simulink model "exercise22_05_"  (R2023b)
settings: Solver=VariableStepAuto  StartTime=0.0  StopTime=30  RelTol=1e-3
libraries: simulink x1
settings Model: Creator=felip  LastModifiedBy=felip

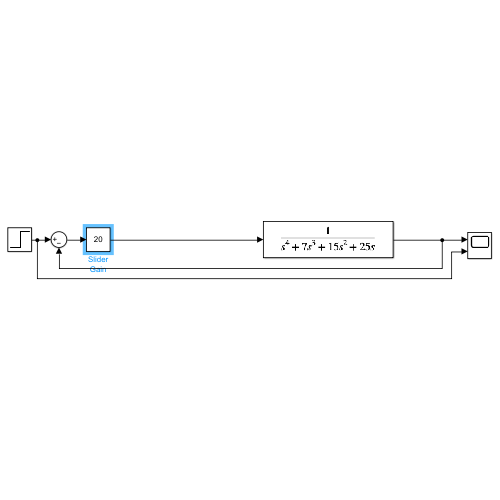
[thumbnail: Simulink's stored preview of the top-level diagram]
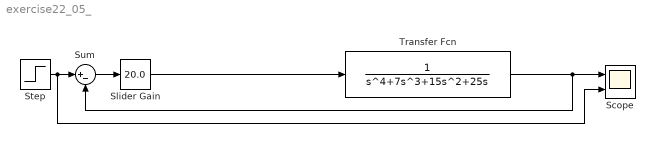
== system exercise22_05_ ==
  Scope : Scope  NumInputPorts=2
  Slider Gain : simulink/Math Operations/Slider Gain  gain=20.0  low=0  high=50
  Step : Step  SampleTime=0
  Sum : Sum  Inputs=|+-
  Transfer Fcn : TransferFcn  Denominator=[1 7 15 25 0]
  wires:
  Transfer Fcn/1 -> Scope/1, Sum/2
  Step/1 -> Scope/2, Sum/1
  Sum/1 -> Slider Gain/1
  Slider Gain/1 -> Transfer Fcn/1
